simulink model "b_r309c_med"  (Simulink 6.2)
settings: Solver=ode45  StartTime=0.0  StopTime=1030.0  RelTol=1e-3
undefined symbols (not defined in the file): ant_bits, BEE2_usr, blockCountBits, blockRowBits, cmult_4bit_em
libraries: xbsIndex_r3 x2808, xps_library x97, casper_library x84
(part 9 of 20)

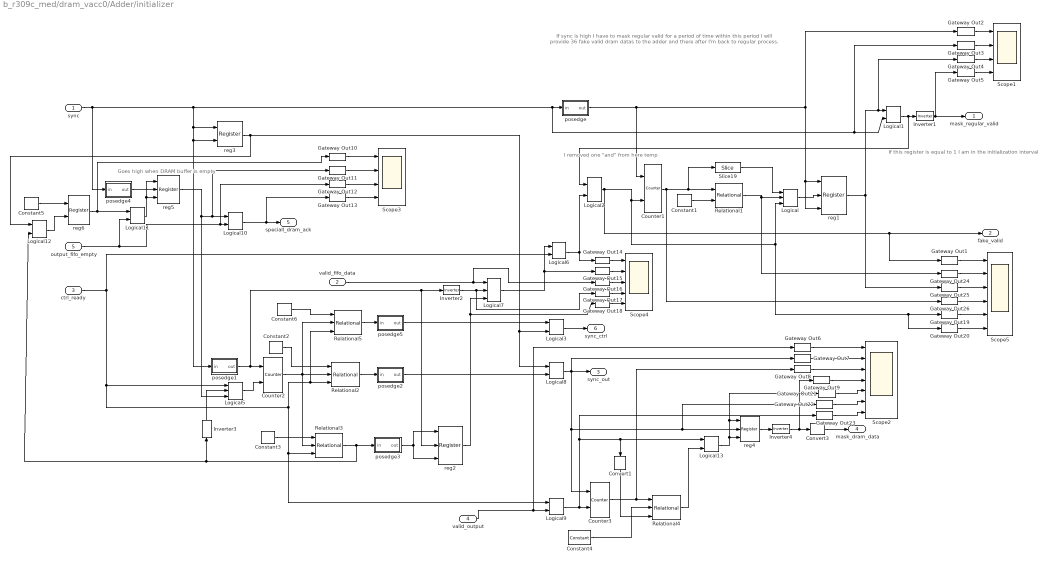
== system b_r309c_med/dram_vacc0/Adder/initializer ==
  note: I removed one "and"
      | from here temp
  note: If this register is equal to 1 I am
      | in the initialization interval
  note: If sync is high I have to mask regular valid for a period of time
      | within this period I will provide 36 fake valid dram datas to the adder and there after I'm back to
      | regular process.
  note: Goes high when DRAM
      | buffer is empty
  sync : Inport  Port=1  LatchInput=off
  valid_fifo_data : Inport  Port=2  LatchInput=off
  ctrl_ready : Inport  Port=3  LatchInput=off
  valid_output : Inport  Port=4  LatchInput=off
  output_fifo_empty : Inport  Port=5  LatchInput=off
  Constant1 : xbsIndex_r3/Constant  const=34  equ=P=C  arith_type=Unsigned  n_bits=6  bin_pt=0  opselect=C  inp2=PCIN>>17  opr=+  inp1=P  carry=CIN  iostate=0  explicit_period=on  period=1  dbl_ovrd=off
  Constant2 : xbsIndex_r3/Constant  const=7  equ=P=C  arith_type=Unsigned  n_bits=4  bin_pt=0  opselect=C  inp2=PCIN>>17  opr=+  inp1=P  carry=CIN  iostate=0  explicit_period=on  period=1  dbl_ovrd=off
  Constant3 : xbsIndex_r3/Constant  const=14  equ=P=C  arith_type=Unsigned  n_bits=4  bin_pt=0  opselect=C  inp2=PCIN>>17  opr=+  inp1=P  carry=CIN  iostate=0  explicit_period=on  period=1  dbl_ovrd=off
  Constant4 : xbsIndex_r3/Constant  const=acc_length-2  equ=P=C  arith_type=Unsigned  n_bits=22  bin_pt=0  opselect=C  inp2=PCIN>>17  opr=+  inp1=P  carry=CIN  iostate=0  explicit_period=on  period=1  dbl_ovrd=off
  Constant5 : xbsIndex_r3/Constant  const=0  equ=P=C  arith_type=Boolean  n_bits=4  bin_pt=0  opselect=C  inp2=PCIN>>17  opr=+  inp1=P  carry=CIN  iostate=0  explicit_period=on  period=1  dbl_ovrd=off
  Constant6 : xbsIndex_r3/Constant  const=4  equ=P=C  arith_type=Unsigned  n_bits=4  bin_pt=0  opselect=C  inp2=PCIN>>17  opr=+  inp1=P  carry=CIN  iostate=0  explicit_period=on  period=1  dbl_ovrd=off
  Convert1 : xbsIndex_r3/Convert  Orientation=down  arith_type=Boolean  n_bits=1  bin_pt=0  quantization=Truncate  overflow=Wrap  latency=0  explicit_period=off  period=1  dbl_ovrd=off  show_param=off  inserted_by_tool=off  pipeline=off
      settings: xl_area=[0, 0, 0, 0, 0, 0, 0]
  Convert3 : xbsIndex_r3/Convert  arith_type=Unsigned  n_bits=1  bin_pt=0  quantization=Truncate  overflow=Wrap  latency=0  explicit_period=off  period=1  dbl_ovrd=off  show_param=off  inserted_by_tool=off  pipeline=off
      settings: xl_area=[0, 0, 0, 0, 0, 0, 0]
  Counter1 : xbsIndex_r3/Counter  cnt_type=Count Limited  n_bits=6  bin_pt=0  arith_type=Unsigned  start_count=0  cnt_to=35  cnt_by_val=1  operation=Up  explicit_period=on  period=1  load_pin=off  rst=on  en=on  dbl_ovrd=off  show_param=off  use_rpm=on  gen_core=off
      settings: xl_area=[0, 0, 0, 0, 0, 0, 0]
  Counter2 : xbsIndex_r3/Counter  cnt_type=Free Running  n_bits=4  bin_pt=0  arith_type=Unsigned  start_count=0  cnt_to=35  cnt_by_val=1  operation=Up  explicit_period=on  period=1  load_pin=off  rst=on  en=on  dbl_ovrd=off  show_param=off  use_rpm=on  gen_core=off
      settings: xl_area=[0, 0, 0, 0, 0, 0, 0]
  Counter3 : xbsIndex_r3/Counter  cnt_type=Free Running  n_bits=22  bin_pt=0  arith_type=Unsigned  start_count=0  cnt_to=35  cnt_by_val=1  operation=Up  explicit_period=on  period=1  load_pin=off  rst=on  en=on  dbl_ovrd=off  show_param=off  use_rpm=on  gen_core=off
      settings: xl_area=[0, 0, 0, 0, 0, 0, 0]
  Gateway Out{1..26} (26 alike) : xbsIndex_r3/Gateway Out  output_type=Double  nbits=8  bin_pt=6  arith_type=Boolean  quantization=Truncate  overflow=Wrap  hdl_port=off  timing_constraint=None  locs_specified=off  LOCs={}  needs_fixed_name=off  show_param=off
      settings: xl_area=[0, 0, 0, 0, 0, 0, 0]
  Inverter1 : xbsIndex_r3/Inverter  latency=0  explicit_period=off  period=1  en=off  dbl_ovrd=off  show_param=off
      settings: xl_area=[0, 0, 0, 0, 0, 0, 0]
  Inverter2 : xbsIndex_r3/Inverter  latency=0  explicit_period=off  period=1  en=off  dbl_ovrd=off  show_param=off
      settings: xl_area=[0, 0, 0, 0, 0, 0, 0]
  Inverter3 : xbsIndex_r3/Inverter  Orientation=up  latency=0  explicit_period=off  period=1  en=off  dbl_ovrd=off  show_param=off
      settings: xl_area=[0, 0, 0, 0, 0, 0, 0]
  Inverter4 : xbsIndex_r3/Inverter  latency=0  explicit_period=off  period=1  en=off  dbl_ovrd=off  show_param=off
      settings: xl_area=[0, 0, 0, 0, 0, 0, 0]
  Logical : xbsIndex_r3/Logical  logical_function=AND  inputs=3  precision=Full  arith_type=Unsigned  n_bits=8  bin_pt=2  align_bp=on  latency=0  explicit_period=on  period=1  en=off  dbl_ovrd=off  show_param=off
      settings: xl_area=[0, 0, 0, 0, 0, 0, 0]
  Logical1 : xbsIndex_r3/Logical  logical_function=OR  inputs=2  precision=Full  arith_type=Unsigned  n_bits=8  bin_pt=2  align_bp=on  latency=0  explicit_period=off  period=1  en=off  dbl_ovrd=off  show_param=off
      settings: xl_area=[0, 0, 0, 0, 0, 0, 0]
  Logical10 : xbsIndex_r3/Logical  logical_function=NOR  inputs=2  precision=Full  arith_type=Unsigned  n_bits=8  bin_pt=2  align_bp=on  latency=0  explicit_period=off  period=1  en=off  dbl_ovrd=off  show_param=off
      settings: xl_area=[0, 0, 0, 0, 0, 0, 0]
  Logical11 : xbsIndex_r3/Logical  logical_function=OR  inputs=2  precision=Full  arith_type=Unsigned  n_bits=8  bin_pt=2  align_bp=on  latency=0  explicit_period=off  period=1  en=off  dbl_ovrd=off  show_param=off
      settings: xl_area=[0, 0, 0, 0, 0, 0, 0]
  Logical{2..3,6,8..9,12..13} (7 alike) : xbsIndex_r3/Logical  logical_function=AND  inputs=2  precision=Full  arith_type=Unsigned  n_bits=8  bin_pt=2  align_bp=on  latency=0  explicit_period=off  period=1  en=off  dbl_ovrd=off  show_param=off
      settings: xl_area=[0, 0, 0, 0, 0, 0, 0]
  Logical5 : xbsIndex_r3/Logical  logical_function=AND  inputs=3  precision=Full  arith_type=Unsigned  n_bits=8  bin_pt=2  align_bp=on  latency=0  explicit_period=off  period=1  en=off  dbl_ovrd=off  show_param=off
      settings: xl_area=[0, 0, 0, 0, 0, 0, 0]
  Logical7 : xbsIndex_r3/Logical  logical_function=AND  inputs=3  precision=Full  arith_type=Unsigned  n_bits=8  bin_pt=2  align_bp=on  latency=0  explicit_period=off  period=1  en=off  dbl_ovrd=off  show_param=off
      settings: xl_area=[0, 0, 0, 0, 0, 0, 0]
  Relational1 : xbsIndex_r3/Relational  mode=a>=b  latency=1  explicit_period=on  period=1  en=off  dbl_ovrd=off  show_param=off
      settings: xl_area=[0, 0, 0, 0, 0, 0, 0]
  Relational2 : xbsIndex_r3/Relational  mode=a<=b  latency=1  explicit_period=on  period=1  en=on  dbl_ovrd=off  show_param=off
      settings: xl_area=[0, 0, 0, 0, 0, 0, 0]
  Relational3 : xbsIndex_r3/Relational  mode=a<=b  latency=1  explicit_period=on  period=1  en=on  dbl_ovrd=off  show_param=off
      settings: xl_area=[0, 0, 0, 0, 0, 0, 0]
  Relational4 : xbsIndex_r3/Relational  mode=a=b  latency=1  explicit_period=on  period=1  en=on  dbl_ovrd=off  show_param=off
      settings: xl_area=[0, 0, 0, 0, 0, 0, 0]
  Relational5 : xbsIndex_r3/Relational  mode=a<=b  latency=1  explicit_period=on  period=1  en=on  dbl_ovrd=off  show_param=off
      settings: xl_area=[0, 0, 0, 0, 0, 0, 0]
  Scope1 : Scope  NumInputPorts=4
      settings: YMin=-1~-1~50~0  YMax=1~1~90~1  SaveName=ScopeData13
  Scope2 : Scope  NumInputPorts=7
      settings: YMin=-1~-1~50~0~-5~-5~-5  YMax=1~1~90~1~5~5~5  SaveName=ScopeData15
  Scope3 : Scope  NumInputPorts=4
      settings: YMin=-1~-1~50~0  YMax=1~1~90~1  SaveName=ScopeData18
  Scope4 : Scope  NumInputPorts=5
      settings: YMin=-1~-1~50~0~-5  YMax=1~1~90~1~5  SaveName=ScopeData31
  Scope5 : Scope  NumInputPorts=6
      settings: YMin=-1~-1~50~0~-5~-5  YMax=1~1~90~1~5~5  SaveName=ScopeData3
  Slice19 : xbsIndex_r3/Slice  mode=Lower Bit Location + Width  nbits=1  bit1=0  base1=MSB of Input  bit0=0  base0=LSB of Input  boolean_output=on  explicit_period=off  period=1  dbl_ovrd=off
  posedge : Subsystem
  posedge1 : Subsystem
  posedge2 : Subsystem
  posedge3 : Subsystem
  posedge4 : Subsystem
  posedge5 : Subsystem
  reg{1..2,4..5} (4 alike) : xbsIndex_r3/Register  init=0  reg_only_valid=off  explicit_period=on  period=1  rst=on  en=on  out_en=off  dbl_ovrd=off  show_param=off
      settings: xl_area=[0, 0, 0, 0, 0, 0, 0]
  reg3 : xbsIndex_r3/Register  init=0  reg_only_valid=off  explicit_period=on  period=1  rst=off  en=on  out_en=off  dbl_ovrd=off  show_param=off
      settings: xl_area=[0, 0, 0, 0, 0, 0, 0]
  reg6 : xbsIndex_r3/Register  init=1  reg_only_valid=off  explicit_period=on  period=1  rst=off  en=on  out_en=off  dbl_ovrd=off  show_param=off
      settings: xl_area=[0, 0, 0, 0, 0, 0, 0]
  mask_regular_valid : Outport
  fake_valid : Outport  Port=2
  sync_out : Outport  Port=3
  mask_dram_data : Outport  Port=4
  speciall_dram_ack : Outport  Port=5
  sync_ctrl : Outport  Port=6
  wires:
  Convert1/1 -> Relational4/3
  Gateway Out23/1 -> Scope2/7
  Gateway Out22/1 -> Scope2/6
  Gateway Out21/1 -> Scope2/5
  Slice19/1 -> Logical/1
  Gateway Out20/1 -> Scope5/6
  Gateway Out19/1 -> Scope5/5
  Gateway Out18/1 -> Scope4/5
  Gateway Out17/1 -> Scope4/4
  Gateway Out16/1 -> Scope4/3
  Gateway Out15/1 -> Scope4/2
  Gateway Out14/1 -> Scope4/1
  Convert3/1 -> mask_dram_data/1
  Relational4/1 -> Logical13/2
  Logical13/1 -> Gateway Out21/1, reg4/1, reg4/3
  reg6/1 -> Gateway Out10/1, Logical11/1
  Logical12/1 -> reg6/2
  Constant5/1 -> reg6/1
  Gateway Out10/1 -> Scope3/1
  Gateway Out13/1 -> Scope3/4
  Gateway Out12/1 -> Scope3/3
  Gateway Out11/1 -> Scope3/2
  Logical11/1 -> reg5/3, reg5/1
  Logical10/1 -> Gateway Out13/1, speciall_dram_ack/1
  output_fifo_empty/1 -> Gateway Out12/1, Logical10/2, Logical11/2
  reg5/1 -> Gateway Out11/1, Logical10/1, Logical5/3
  posedge4/1(out) -> reg5/2
  Gateway Out6/1 -> Scope2/1
  Gateway Out9/1 -> Scope2/4
  Gateway Out8/1 -> Scope2/3
  Gateway Out7/1 -> Scope2/2
  Inverter4/1 -> Convert3/1, Gateway Out9/1
  reg4/1 -> Inverter4/1
  Constant4/1 -> Relational4/2
  Counter3/1 -> Gateway Out8/1, Relational4/1
  valid_output/1 -> Gateway Out6/1, Logical9/2
  Logical9/1 -> Convert1/1, Logical13/1, Gateway Out23/1, Counter3/2
  reg3/1 -> Logical12/1, Logical8/1, Logical3/2
  posedge2/1(out) -> Logical8/2
  Logical8/1 -> Gateway Out7/1, Gateway Out22/1, reg4/2, Counter3/1, sync_out/1
  Inverter3/1 -> Logical5/2
  Logical5/1 -> Counter2/2
  Logical7/1 -> Gateway Out15/1, Logical6/1
  valid_fifo_data/1 -> Gateway Out16/1, Logical7/1
  Inverter2/1 -> Gateway Out17/1, Logical7/2
  reg2/1 -> Gateway Out18/1, Logical7/3
  posedge3/1(out) -> reg2/3, reg2/1
  Relational3/1 -> Logical12/2, Inverter3/1, posedge3/1(in)
  Constant3/1 -> Relational3/1
  Relational2/1 -> posedge2/1(in)
  Constant2/1 -> Relational2/1
  Counter2/1 -> Relational3/2, Relational2/2, Relational5/2
  posedge1/1(out) -> Inverter2/1, reg2/2, Counter2/1
  Inverter1/1 -> Gateway Out5/1, mask_regular_valid/1
  Logical/1 -> reg1/2
  Logical6/1 -> Gateway Out14/1, Logical2/2
  ctrl_ready/1 -> Logical9/1, Relational3/3, Relational2/3, Relational5/3, Logical5/1, Logical6/2
  Relational1/1 -> Logical/2, Gateway Out24/1
  reg1/1 -> Gateway Out25/1, Gateway Out4/1, Logical1/1
  Constant1/1 -> Relational1/2
  Counter1/1 -> Slice19/1, Relational1/1, Gateway Out26/1
  Logical2/1 -> Counter1/2, Gateway Out20/1, Gateway Out19/1, Logical/3, Gateway Out1/1, fake_valid/1
  Logical1/1 -> Logical2/1, Inverter1/1
  posedge/1(out) -> Counter1/1, reg1/3, reg1/1, Gateway Out2/1
  sync/1 -> posedge4/1(in), reg3/1, reg3/2, posedge1/1(in), Gateway Out3/1, Logical1/2, posedge/1(in)
  Gateway Out2/1 -> Scope1/1
  Gateway Out5/1 -> Scope1/4
  Gateway Out4/1 -> Scope1/3
  Gateway Out3/1 -> Scope1/2
  Gateway Out1/1 -> Scope5/1
  Gateway Out26/1 -> Scope5/4
  Gateway Out25/1 -> Scope5/3
  Gateway Out24/1 -> Scope5/2
  Constant6/1 -> Relational5/1
  Relational5/1 -> posedge5/1(in)
  posedge5/1(out) -> Logical3/1
  Logical3/1 -> sync_ctrl/1

== system b_r309c_med/dram_vacc0/RB_reg/Trickle_FWFT ==
  note: We needed a FIFO which brings the valid data automatically to the output.
      | The regular XILINX Fifos are not FWFT (First Word Fall Through).
      | We tried to make one but it was really hard to make one agreeing with the exact specs.
      | This module which we have named it Trickle_FWFT Fifo works very similiarly with minor
      | differences which servers our purpose here in the DRAM VACC module.
  note: The real depth of this module is depth+1.
      | The valid signal will go high with one cycle delay.
  din : Inport  Port=1  LatchInput=off
  we : Inport  Port=2  LatchInput=off
  ack : Inport  Port=3  LatchInput=off
  reset : Inport  Port=4  LatchInput=off
  Convert : xbsIndex_r3/Convert  Orientation=left  arith_type=Boolean  n_bits=8  bin_pt=6  quantization=Truncate  overflow=Wrap  latency=0  explicit_period=on  period=1  dbl_ovrd=off  show_param=off  inserted_by_tool=off  pipeline=off
      settings: xl_area=[0, 0, 0, 0, 0, 0, 0]
  Convert3 : xbsIndex_r3/Convert  arith_type=Boolean  n_bits=8  bin_pt=6  quantization=Truncate  overflow=Wrap  latency=0  explicit_period=off  period=1  dbl_ovrd=off  show_param=off  inserted_by_tool=off  pipeline=off
      settings: xl_area=[0, 0, 0, 0, 0, 0, 0]
  FIFO : xbsIndex_r3/FIFO  depth=16  percent_nbits=1  store_only_valid=on  init_zero=on  explicit_period=on  period=1  rst=on  en=off  use_almost_empty=off  almost_empty_offset=6  use_almost_full=off  almost_full_offset=6  dbl_ovrd=off  show_param=off  mem_type=Block RAM  gen_core=off
      settings: xl_area=[0, 0, 0, 0, 0, 0, 0]
  Inverter3 : xbsIndex_r3/Inverter  latency=0  explicit_period=off  period=1  en=off  dbl_ovrd=off  show_param=off
      settings: xl_area=[0, 0, 0, 0, 0, 0, 0]
  Logical2 : xbsIndex_r3/Logical  logical_function=OR  inputs=2  precision=Full  arith_type=Unsigned  n_bits=8  bin_pt=2  align_bp=on  latency=0  explicit_period=on  period=1  en=off  dbl_ovrd=off  show_param=off
      settings: xl_area=[0, 0, 0, 0, 0, 0, 0]
  not_valid : xbsIndex_r3/Register  init=1  reg_only_valid=off  explicit_period=on  period=1  rst=on  en=on  out_en=off  dbl_ovrd=off  show_param=off
      settings: xl_area=[0, 0, 0, 0, 0, 0, 0]
  data_out : Outport
  valid : Outport  Port=2
  full : Outport  Port=3
  %full : Outport  Port=4
  wires:
  din/1 -> FIFO/1
  we/1 -> FIFO/2
  FIFO/2 -> not_valid/1
  ack/1 -> Logical2/2
  FIFO/1 -> data_out/1
  FIFO/4 -> full/1
  Inverter3/1 -> Convert3/1
  reset/1 -> FIFO/4, not_valid/2
  Logical2/1 -> FIFO/3, not_valid/3
  not_valid/1 -> Inverter3/1, Convert/1
  Convert/1 -> Logical2/1
  FIFO/3 -> %full/1
  Convert3/1 -> valid/1

== system b_r309c_med/dram_vacc0/RB_reg/posedge ==
  in : Inport  Port=1  LatchInput=off
  Delay : xbsIndex_r3/Delay  latency=1  reg_retiming=off  explicit_period=off  period=1  en=off  accept_only_valid=off  init_zero=on  dbl_ovrd=off  show_param=off
      settings: xl_area=[0, 0, 0, 0, 0, 0, 0]
  Inverter2 : xbsIndex_r3/Inverter  latency=0  explicit_period=off  period=1  en=off  dbl_ovrd=off  show_param=off
      settings: xl_area=[0, 0, 0, 0, 0, 0, 0]
  Logical : xbsIndex_r3/Logical  logical_function=AND  inputs=2  precision=Full  arith_type=Unsigned  n_bits=8  bin_pt=2  align_bp=on  latency=0  explicit_period=off  period=1  en=off  dbl_ovrd=off  show_param=off
      settings: xl_area=[0, 0, 0, 0, 0, 0, 0]
  out : Outport
  wires:
  Inverter2/1 -> Logical/1
  Logical/1 -> out/1
  in/1 -> Logical/2, Delay/1
  Delay/1 -> Inverter2/1

== system b_r309c_med/dram_vacc0/ctrl_unit/RB_active_or_finish ==
  enable_rb_addr : Inport  Orientation=down  Port=1  LatchInput=off
  sync : Inport  Port=2  LatchInput=off
  Constant3 : xbsIndex_r3/Constant  const=acc_length/2  equ=P=C  arith_type=Unsigned  n_bits=32  bin_pt=0  opselect=C  inp2=PCIN>>17  opr=+  inp1=P  carry=CIN  iostate=0  explicit_period=on  period=1  dbl_ovrd=off
  Counter1 : xbsIndex_r3/Counter  cnt_type=Free Running  n_bits=32  bin_pt=0  arith_type=Unsigned  start_count=0  cnt_to=2*burst_length-1  cnt_by_val=1  operation=Up  explicit_period=on  period=1  load_pin=off  rst=on  en=on  dbl_ovrd=off  show_param=off  use_rpm=on  gen_core=off
      settings: xl_area=[0, 0, 0, 0, 0, 0, 0]
  Inverter6 : xbsIndex_r3/Inverter  latency=0  explicit_period=off  period=1  en=off  dbl_ovrd=off  show_param=off
      settings: xl_area=[0, 0, 0, 0, 0, 0, 0]
  Inverter9 : xbsIndex_r3/Inverter  latency=0  explicit_period=off  period=1  en=off  dbl_ovrd=off  show_param=off
      settings: xl_area=[0, 0, 0, 0, 0, 0, 0]
  Logical13 : xbsIndex_r3/Logical  logical_function=AND  inputs=3  precision=Full  arith_type=Unsigned  n_bits=8  bin_pt=2  align_bp=on  latency=0  explicit_period=on  period=1  en=off  dbl_ovrd=off  show_param=off
      settings: xl_area=[0, 0, 0, 0, 0, 0, 0]
  Logical14 : xbsIndex_r3/Logical  logical_function=AND  inputs=2  precision=Full  arith_type=Unsigned  n_bits=8  bin_pt=2  align_bp=on  latency=0  explicit_period=on  period=1  en=off  dbl_ovrd=off  show_param=off
      settings: xl_area=[0, 0, 0, 0, 0, 0, 0]
  Logical7 : xbsIndex_r3/Logical  logical_function=AND  inputs=2  precision=Full  arith_type=Unsigned  n_bits=8  bin_pt=2  align_bp=on  latency=0  explicit_period=on  period=1  en=off  dbl_ovrd=off  show_param=off
      settings: xl_area=[0, 0, 0, 0, 0, 0, 0]
  Relational3 : xbsIndex_r3/Relational  mode=a=b  latency=1  explicit_period=on  period=1  en=off  dbl_ovrd=off  show_param=off
      settings: xl_area=[0, 0, 0, 0, 0, 0, 0]
  system_start : xbsIndex_r3/Register  init=0  reg_only_valid=off  explicit_period=off  period=1  rst=off  en=on  out_en=off  dbl_ovrd=off  show_param=off
      settings: xl_area=[0, 0, 0, 0, 0, 0, 0]
  system_start1 : xbsIndex_r3/Register  init=0  reg_only_valid=off  explicit_period=off  period=1  rst=off  en=on  out_en=off  dbl_ovrd=off  show_param=off
      settings: xl_area=[0, 0, 0, 0, 0, 0, 0]
  system_start2 : xbsIndex_r3/Register  init=0  reg_only_valid=off  explicit_period=off  period=1  rst=on  en=on  out_en=off  dbl_ovrd=off  show_param=off
      settings: xl_area=[0, 0, 0, 0, 0, 0, 0]
  rb_active : Outport
  wires:
  Logical13/1 -> rb_active/1
  sync/1 -> system_start2/2, Counter1/1, system_start/2, system_start/1, Logical14/1, Inverter9/1
  enable_rb_addr/1 -> Logical7/1, Counter1/2
  Inverter9/1 -> Logical13/3
  system_start1/1 -> Logical13/2
  Logical14/1 -> system_start1/2, system_start1/1
  Inverter6/1 -> Logical13/1
  Relational3/1 -> Logical7/2
  Logical7/1 -> system_start2/3, system_start2/1
  Constant3/1 -> Relational3/2
  Counter1/1 -> Relational3/1
  system_start2/1 -> Inverter6/1
  system_start/1 -> Logical14/2

== system b_r309c_med/dram_vacc0/ctrl_unit/address_gen_vacc_DRAM ==
  sync : Inport  Port=1  LatchInput=off
  read_en : Inport  Port=2  LatchInput=off
  write_en : Inport  Port=3  LatchInput=off
  and0 : xbsIndex_r3/Logical  logical_function=AND  inputs=2  precision=Full  arith_type=Unsigned  n_bits=8  bin_pt=2  align_bp=on  latency=0  explicit_period=off  period=1  en=off  dbl_ovrd=off  show_param=off
      settings: xl_area=[0, 0, 0, 0, 0, 0, 0]
  block_counter : xbsIndex_r3/Counter  cnt_type=Free Running  n_bits=blockCountBits  bin_pt=0  arith_type=Unsigned  start_count=2^blockCountBits-1  cnt_to=Inf  cnt_by_val=1  operation=Up  explicit_period=off  period=1  load_pin=off  rst=off  en=on  dbl_ovrd=off  show_param=off  use_rpm=on  gen_core=off
      settings: xl_area=[0, 0, 0, 0, 0, 0, 0]
  cast0 : xbsIndex_r3/Convert  arith_type=Unsigned  n_bits=8  bin_pt=0  quantization=Truncate  overflow=Wrap  latency=0  explicit_period=off  period=1  dbl_ovrd=off  show_param=off  inserted_by_tool=off  pipeline=off
      settings: xl_area=[0, 0, 0, 0, 0, 0, 0]
  cast1 : xbsIndex_r3/Convert  arith_type=Unsigned  n_bits=8  bin_pt=0  quantization=Truncate  overflow=Wrap  latency=0  explicit_period=off  period=1  dbl_ovrd=off  show_param=off  inserted_by_tool=off  pipeline=off
      settings: xl_area=[0, 0, 0, 0, 0, 0, 0]
  compare : xbsIndex_r3/Relational  mode=a=b  latency=1  explicit_period=off  period=1  en=off  dbl_ovrd=off  show_param=off
      settings: xl_area=[0, 0, 0, 0, 0, 0, 0]
  compare1 : xbsIndex_r3/Relational  mode=a=b  latency=1  explicit_period=on  period=1  en=off  dbl_ovrd=off  show_param=off
      settings: xl_area=[0, 0, 0, 0, 0, 0, 0]
  concat0 : xbsIndex_r3/Concat  num_inputs=2  explicit_period=off  period=1  dbl_ovrd=off
  concat1 : xbsIndex_r3/Concat  num_inputs=2  explicit_period=off  period=1  dbl_ovrd=off
  concat2 : xbsIndex_r3/Concat  num_inputs=7  explicit_period=off  period=1  dbl_ovrd=off
  concat3 : xbsIndex_r3/Concat  num_inputs=7  explicit_period=off  period=1  dbl_ovrd=off
  const0 : xbsIndex_r3/Constant  const=0  equ=P=C  arith_type=Unsigned  n_bits=5  bin_pt=0  opselect=C  inp2=PCIN>>17  opr=+  inp1=P  carry=CIN  iostate=0  explicit_period=off  period=1  dbl_ovrd=off
  const1 : xbsIndex_r3/Constant  const=0  equ=P=C  arith_type=Unsigned  n_bits=2  bin_pt=0  opselect=C  inp2=PCIN>>17  opr=+  inp1=P  carry=CIN  iostate=0  explicit_period=off  period=1  dbl_ovrd=off
  const10 : xbsIndex_r3/Constant  const=valid_length/2  equ=P=C  arith_type=Unsigned  n_bits=counterBitWidth  bin_pt=0  opselect=C  inp2=PCIN>>17  opr=+  inp1=P  carry=CIN  iostate=0  explicit_period=on  period=1  dbl_ovrd=off
  const11 : xbsIndex_r3/Constant  const=acc_length/2-1  equ=P=C  arith_type=Unsigned  n_bits=counterBitWidth  bin_pt=0  opselect=C  inp2=PCIN>>17  opr=+  inp1=P  carry=CIN  iostate=0  explicit_period=on  period=1  dbl_ovrd=off
  const4 : xbsIndex_r3/Constant  const=acc_length/2-1  equ=P=C  arith_type=Unsigned  n_bits=counterBitWidth  bin_pt=0  opselect=C  inp2=PCIN>>17  opr=+  inp1=P  carry=CIN  iostate=0  explicit_period=off  period=1  dbl_ovrd=off
  or0 : xbsIndex_r3/Logical  logical_function=OR  inputs=2  precision=Full  arith_type=Unsigned  n_bits=8  bin_pt=2  align_bp=on  latency=0  explicit_period=off  period=1  en=off  dbl_ovrd=off  show_param=off
      settings: xl_area=[0, 0, 0, 0, 0, 0, 0]
  read_counter : xbsIndex_r3/Counter  cnt_type=Free Running  n_bits=counterBitWidth  bin_pt=0  arith_type=Unsigned  start_count=0  cnt_to=Inf  cnt_by_val=1  operation=Up  explicit_period=off  period=1  load_pin=on  rst=on  en=on  dbl_ovrd=off  show_param=off  use_rpm=on  gen_core=off
      settings: xl_area=[0, 0, 0, 0, 0, 0, 0]
  slice0 : xbsIndex_r3/Slice  mode=Lower Bit Location + Width  nbits=colCountBits  bit1=0  base1=MSB of Input  bit0=0  base0=LSB of Input  boolean_output=off  explicit_period=off  period=1  dbl_ovrd=off
  slice1 : xbsIndex_r3/Slice  mode=Upper Bit Location + Width  nbits=blockCountBits+blockRowBits  bit1=0  base1=MSB of Input  bit0=0  base0=LSB of Input  boolean_output=off  explicit_period=off  period=1  dbl_ovrd=off
  slice10 : xbsIndex_r3/Slice  mode=Lower Bit Location + Width  nbits=2  bit1=0  base1=MSB of Input  bit0=0  base0=LSB of Input  boolean_output=off  explicit_period=off  period=1  dbl_ovrd=off
  slice11 : xbsIndex_r3/Slice  mode=Upper Bit Location + Width  nbits=blockCountBits-2  bit1=0  base1=MSB of Input  bit0=0  base0=LSB of Input  boolean_output=off  explicit_period=off  period=1  dbl_ovrd=off
  slice12 : xbsIndex_r3/Slice  mode=Upper Bit Location + Width  nbits=1  bit1=0  base1=MSB of Input  bit0=0  base0=LSB of Input  boolean_output=off  explicit_period=off  period=1  dbl_ovrd=off
  slice13 : xbsIndex_r3/Slice  mode=Lower Bit Location + Width  nbits=blockCountBits-3  bit1=0  base1=MSB of Input  bit0=0  base0=LSB of Input  boolean_output=off  explicit_period=off  period=1  dbl_ovrd=off
  slice14 : xbsIndex_r3/Slice  mode=Upper Bit Location + Width  nbits=1  bit1=0  base1=MSB of Input  bit0=0  base0=LSB of Input  boolean_output=off  explicit_period=off  period=1  dbl_ovrd=off
  slice15 : xbsIndex_r3/Slice  mode=Lower Bit Location + Width  nbits=blockCountBits-3  bit1=0  base1=MSB of Input  bit0=0  base0=LSB of Input  boolean_output=off  explicit_period=off  period=1  dbl_ovrd=off
  slice2 : xbsIndex_r3/Slice  mode=Lower Bit Location + Width  nbits=blockRowBits  bit1=0  base1=MSB of Input  bit0=0  base0=LSB of Input  boolean_output=off  explicit_period=off  period=1  dbl_ovrd=off
  slice3 : xbsIndex_r3/Slice  mode=Upper Bit Location + Width  nbits=blockCountBits  bit1=0  base1=MSB of Input  bit0=0  base0=LSB of Input  boolean_output=off  explicit_period=off  period=1  dbl_ovrd=off
  slice4 : xbsIndex_r3/Slice  mode=Lower Bit Location + Width  nbits=2  bit1=0  base1=MSB of Input  bit0=0  base0=LSB of Input  boolean_output=off  explicit_period=off  period=1  dbl_ovrd=off
  slice5 : xbsIndex_r3/Slice  mode=Upper Bit Location + Width  nbits=blockCountBits-2  bit1=0  base1=MSB of Input  bit0=0  base0=LSB of Input  boolean_output=off  explicit_period=off  period=1  dbl_ovrd=off
  slice6 : xbsIndex_r3/Slice  mode=Lower Bit Location + Width  nbits=colCountBits  bit1=0  base1=MSB of Input  bit0=0  base0=LSB of Input  boolean_output=off  explicit_period=off  period=1  dbl_ovrd=off
  slice7 : xbsIndex_r3/Slice  mode=Upper Bit Location + Width  nbits=blockCountBits+blockRowBits  bit1=0  base1=MSB of Input  bit0=0  base0=LSB of Input  boolean_output=off  explicit_period=off  period=1  dbl_ovrd=off
  slice8 : xbsIndex_r3/Slice  mode=Lower Bit Location + Width  nbits=blockRowBits  bit1=0  base1=MSB of Input  bit0=0  base0=LSB of Input  boolean_output=off  explicit_period=off  period=1  dbl_ovrd=off
  slice9 : xbsIndex_r3/Slice  mode=Upper Bit Location + Width  nbits=blockCountBits  bit1=0  base1=MSB of Input  bit0=0  base0=LSB of Input  boolean_output=off  explicit_period=off  period=1  dbl_ovrd=off
  write_counter : xbsIndex_r3/Counter  cnt_type=Count Limited  n_bits=counterBitWidth  bin_pt=0  arith_type=Unsigned  start_count=0  cnt_to=acc_length/2-1  cnt_by_val=1  operation=Up  explicit_period=off  period=1  load_pin=off  rst=on  en=on  dbl_ovrd=off  show_param=off  use_rpm=on  gen_core=off
      settings: xl_area=[0, 0, 0, 0, 0, 0, 0]
  write_addr : Outport
  read_addr : Outport  Port=2
  end_masking : Outport  Port=3
  wires:
  slice1/1 -> slice2/1, slice3/1
  const1/1 -> concat2/1, concat3/1
  slice4/1 -> concat2/2
  slice13/1 -> concat2/3
  slice2/1 -> concat2/4
  slice12/1 -> concat2/5
  cast0/1 -> concat2/6
  const0/1 -> concat2/7, concat3/7
  slice7/1 -> slice8/1, slice9/1
  slice10/1 -> concat3/2
  slice15/1 -> concat3/3
  slice8/1 -> concat3/4
  slice14/1 -> concat3/5
  cast1/1 -> concat3/6
  sync/1 -> write_counter/1, read_counter/1, block_counter/1, or0/1
  const10/1 -> read_counter/2
  write_en/1 -> write_counter/2
  block_counter/1 -> concat0/1, concat1/1
  write_counter/1 -> concat0/2, compare/1
  read_counter/1 -> concat1/2, compare1/1
  const4/1 -> compare/2
  compare/1 -> end_masking/1
  const11/1 -> compare1/2
  concat0/1 -> slice0/1, slice1/1
  slice0/1 -> cast0/1
  slice3/1 -> slice4/1, slice5/1
  concat2/1 -> write_addr/1
  concat1/1 -> slice6/1, slice7/1
  slice6/1 -> cast1/1
  slice9/1 -> slice10/1, slice11/1
  concat3/1 -> read_addr/1
  slice5/1 -> slice12/1, slice13/1
  slice11/1 -> slice14/1, slice15/1
  read_en/1 -> or0/2, and0/1
  or0/1 -> read_counter/4
  compare1/1 -> and0/2
  and0/1 -> read_counter/3

== system b_r309c_med/dram_vacc0/ctrl_unit/cmd_gen ==
  note: Logic here is added to handle an  odd number of input valid datas.
      | In case we receive a new sync and valid_wr_cnt is high, we mask the wr_be
      | signal of DRAM and issue a write command to finish the last command.
  valid_data : Inport  Port=1  LatchInput=off
  sync : Inport  Port=2  LatchInput=off
  Constant : xbsIndex_r3/Constant  const=burst_length-1  equ=P=C  arith_type=Unsigned  n_bits=ceil(log2(2*burst_length+2))  bin_pt=0  opselect=C  inp2=PCIN>>17  opr=+  inp1=P  carry=CIN  iostate=0  explicit_period=on  period=1  dbl_ovrd=off
  Constant1 : xbsIndex_r3/Constant  const=burst_length-1  equ=P=C  arith_type=Unsigned  n_bits=ceil(log2(2*burst_length+2))  bin_pt=0  opselect=C  inp2=PCIN>>17  opr=+  inp1=P  carry=CIN  iostate=0  explicit_period=on  period=1  dbl_ovrd=off
  Constant2 : xbsIndex_r3/Constant  const=2*burst_length+2-1  equ=P=C  arith_type=Unsigned  n_bits=ceil(log2(2*burst_length+2))  bin_pt=0  opselect=C  inp2=PCIN>>17  opr=+  inp1=P  carry=CIN  iostate=0  explicit_period=on  period=1  dbl_ovrd=off
  Constant3 : xbsIndex_r3/Constant  const=2^18-1  equ=P=C  arith_type=Unsigned  n_bits=18  bin_pt=0  opselect=C  inp2=PCIN>>17  opr=+  inp1=P  carry=CIN  iostate=0  explicit_period=on  period=1  dbl_ovrd=off
  Constant4 : xbsIndex_r3/Constant  const=2*burst_length  equ=P=C  arith_type=Unsigned  n_bits=ceil(log2(2*burst_length+2))  bin_pt=0  opselect=C  inp2=PCIN>>17  opr=+  inp1=P  carry=CIN  iostate=0  explicit_period=on  period=1  dbl_ovrd=off
  Convert1 : xbsIndex_r3/Convert  arith_type=Boolean  n_bits=31  bin_pt=0  quantization=Truncate  overflow=Wrap  latency=0  explicit_period=on  period=1  dbl_ovrd=off  show_param=off  inserted_by_tool=off  pipeline=off
      settings: xl_area=[0, 0, 0, 0, 0, 0, 0]
  Delay : xbsIndex_r3/Delay  latency=1  reg_retiming=off  explicit_period=off  period=1  en=on  accept_only_valid=off  init_zero=on  dbl_ovrd=off  show_param=off
      settings: xl_area=[0, 0, 0, 0, 0, 0, 0]
  Delay1 : xbsIndex_r3/Delay  latency=1  reg_retiming=off  explicit_period=off  period=1  en=off  accept_only_valid=off  init_zero=on  dbl_ovrd=off  show_param=off
      settings: xl_area=[0, 0, 0, 0, 0, 0, 0]
  Delay3 : xbsIndex_r3/Delay  latency=1  reg_retiming=off  explicit_period=on  period=1  en=off  accept_only_valid=off  init_zero=on  dbl_ovrd=off  show_param=off
      settings: xl_area=[0, 0, 0, 0, 0, 0, 0]
  Delay4 : xbsIndex_r3/Delay  latency=1  reg_retiming=off  explicit_period=on  period=1  en=off  accept_only_valid=off  init_zero=on  dbl_ovrd=off  show_param=off
      settings: xl_area=[0, 0, 0, 0, 0, 0, 0]
  Inverter{1..5} (5 alike) : xbsIndex_r3/Inverter  latency=0  explicit_period=off  period=1  en=off  dbl_ovrd=off  show_param=off
      settings: xl_area=[0, 0, 0, 0, 0, 0, 0]
  Inverter8 : xbsIndex_r3/Inverter  Orientation=down  latency=0  explicit_period=off  period=1  en=off  dbl_ovrd=off  show_param=off
      settings: xl_area=[0, 0, 0, 0, 0, 0, 0]
  Logical{,2,8..9,12,15} (6 alike) : xbsIndex_r3/Logical  logical_function=AND  inputs=2  precision=Full  arith_type=Unsigned  n_bits=8  bin_pt=2  align_bp=on  latency=0  explicit_period=on  period=1  en=off  dbl_ovrd=off  show_param=off
      settings: xl_area=[0, 0, 0, 0, 0, 0, 0]
  Logical1 : xbsIndex_r3/Logical  logical_function=AND  inputs=3  precision=Full  arith_type=Unsigned  n_bits=8  bin_pt=2  align_bp=on  latency=0  explicit_period=on  period=1  en=off  dbl_ovrd=off  show_param=off
      settings: xl_area=[0, 0, 0, 0, 0, 0, 0]
  Logical10 : xbsIndex_r3/Logical  logical_function=OR  inputs=2  precision=Full  arith_type=Unsigned  n_bits=8  bin_pt=2  align_bp=on  latency=0  explicit_period=on  period=1  en=off  dbl_ovrd=off  show_param=off
      settings: xl_area=[0, 0, 0, 0, 0, 0, 0]
  Logical11 : xbsIndex_r3/Logical  logical_function=OR  inputs=2  precision=Full  arith_type=Unsigned  n_bits=8  bin_pt=2  align_bp=on  latency=0  explicit_period=on  period=1  en=off  dbl_ovrd=off  show_param=off
      settings: xl_area=[0, 0, 0, 0, 0, 0, 0]
  Logical3 : xbsIndex_r3/Logical  logical_function=AND  inputs=3  precision=Full  arith_type=Unsigned  n_bits=8  bin_pt=2  align_bp=on  latency=0  explicit_period=off  period=1  en=off  dbl_ovrd=off  show_param=off
      settings: xl_area=[0, 0, 0, 0, 0, 0, 0]
  Logical4 : xbsIndex_r3/Logical  logical_function=OR  inputs=2  precision=Full  arith_type=Unsigned  n_bits=8  bin_pt=2  align_bp=on  latency=0  explicit_period=off  period=1  en=off  dbl_ovrd=off  show_param=off
      settings: xl_area=[0, 0, 0, 0, 0, 0, 0]
  Logical5 : xbsIndex_r3/Logical  logical_function=OR  inputs=2  precision=Full  arith_type=Unsigned  n_bits=8  bin_pt=2  align_bp=on  latency=0  explicit_period=off  period=1  en=off  dbl_ovrd=off  show_param=off
      settings: xl_area=[0, 0, 0, 0, 0, 0, 0]
  Logical6 : xbsIndex_r3/Logical  logical_function=OR  inputs=2  precision=Full  arith_type=Unsigned  n_bits=8  bin_pt=2  align_bp=on  latency=0  explicit_period=on  period=1  en=off  dbl_ovrd=off  show_param=off
      settings: xl_area=[0, 0, 0, 0, 0, 0, 0]
  Relational : xbsIndex_r3/Relational  mode=a>=b  latency=1  explicit_period=on  period=1  en=on  dbl_ovrd=off  show_param=off
      settings: xl_area=[0, 0, 0, 0, 0, 0, 0]
  Relational1 : xbsIndex_r3/Relational  mode=a<=b  latency=1  explicit_period=on  period=1  en=on  dbl_ovrd=off  show_param=off
      settings: xl_area=[0, 0, 0, 0, 0, 0, 0]
  Relational2 : xbsIndex_r3/Relational  mode=a!=b  latency=1  explicit_period=off  period=1  en=on  dbl_ovrd=off  show_param=off
      settings: xl_area=[0, 0, 0, 0, 0, 0, 0]
  Relational4 : xbsIndex_r3/Relational  mode=a<=b  latency=1  explicit_period=on  period=1  en=on  dbl_ovrd=off  show_param=off
      settings: xl_area=[0, 0, 0, 0, 0, 0, 0]
  Slice : xbsIndex_r3/Slice  mode=Lower Bit Location + Width  nbits=1  bit1=0  base1=MSB of Input  bit0=0  base0=LSB of Input  boolean_output=on  explicit_period=off  period=1  dbl_ovrd=off
  cmd_counter : xbsIndex_r3/Counter  cnt_type=Count Limited  n_bits=ceil(log2(2*burst_length+2))  bin_pt=0  arith_type=Unsigned  start_count=0  cnt_to=2*burst_length+2-1  cnt_by_val=1  operation=Up  explicit_period=on  period=1  load_pin=off  rst=on  en=on  dbl_ovrd=off  show_param=off  use_rpm=on  gen_core=off
      settings: xl_area=[0, 0, 0, 0, 0, 0, 0]
  system_start : xbsIndex_r3/Register  init=0  reg_only_valid=off  explicit_period=off  period=1  rst=off  en=on  out_en=off  dbl_ovrd=off  show_param=off
      settings: xl_area=[0, 0, 0, 0, 0, 0, 0]
  re_addr_en : Outport
  wr_addr_en : Outport  Port=2
  RWn : Outport  Port=3
  cmd_valid : Outport  Port=4
  ready : Outport  Port=5
  rb_addr_en : Outport  Port=6
  wr_be : Outport  Port=7
  wires:
  Logical9/1 -> wr_addr_en/1
  Logical8/1 -> re_addr_en/1
  Logical15/1 -> Logical4/1, Logical11/1
  Inverter8/1 -> Logical1/3
  Relational4/1 -> rb_addr_en/1, Inverter8/1
  Constant4/1 -> Relational4/1
  Logical6/1 -> Delay/2, Relational4/3, Relational/3, Relational1/3, Relational2/3
  Delay4/1 -> Logical6/1, Logical5/2
  Logical5/1 -> cmd_counter/1
  Logical2/1 -> Delay3/1
  Logical12/1 -> Logical2/1
  Convert1/1 -> Logical2/2, Logical8/2, Logical9/2, Logical6/2
  Inverter5/1 -> Logical15/2, ready/1
  Inverter4/1 -> Logical10/1
  Logical10/1 -> Logical12/1
  Inverter3/1 -> RWn/1
  Inverter2/1 -> Logical1/2
  system_start/1 -> Logical12/2
  Logical4/1 -> cmd_counter/2
  Logical3/1 -> Logical11/2, Logical4/2, Inverter5/1
  valid_data/1 -> Logical15/1
  Delay1/1 -> Inverter1/1
  Inverter1/1 -> Logical3/2
  Relational2/1 -> Logical3/3
  Constant2/1 -> Relational2/1
  Relational1/1 -> Logical3/1
  Constant1/1 -> Relational1/1
  Delay/1 -> Logical/1, Logical1/1
  Relational/1 -> Inverter3/1, Logical10/2, Logical/2, Inverter2/1
  Slice/1 -> Inverter4/1, Delay/1
  Logical1/1 -> Logical8/1
  Logical/1 -> Logical9/1
  Logical11/1 -> Convert1/1
  Constant/1 -> Relational/1
  cmd_counter/1 -> Relational2/2, Relational1/2, Relational4/2, Relational/2, Slice/1
  sync/1 -> Delay4/1, Logical5/1, system_start/1, system_start/2, Delay1/1
  Constant3/1 -> wr_be/1
  Delay3/1 -> cmd_valid/1

== system b_r309c_med/dram_vacc0/ctrl_unit/latch_rb_enable ==
  sync : Inport  Port=1  LatchInput=off
  rb_addr_enable : Inport  Port=2  LatchInput=off
  negedge : Inport  Port=3  LatchInput=off
  Inverter5 : xbsIndex_r3/Inverter  latency=0  explicit_period=off  period=1  en=off  dbl_ovrd=off  show_param=off
      settings: xl_area=[0, 0, 0, 0, 0, 0, 0]
  Logical1 : xbsIndex_r3/Logical  logical_function=OR  inputs=2  precision=Full  arith_type=Unsigned  n_bits=8  bin_pt=2  align_bp=on  latency=0  explicit_period=on  period=1  en=off  dbl_ovrd=off  show_param=off
      settings: xl_area=[0, 0, 0, 0, 0, 0, 0]
  Logical2 : xbsIndex_r3/Logical  logical_function=OR  inputs=2  precision=Full  arith_type=Unsigned  n_bits=8  bin_pt=2  align_bp=on  latency=1  explicit_period=on  period=1  en=off  dbl_ovrd=off  show_param=off
      settings: xl_area=[0, 0, 0, 0, 0, 0, 0]
  Logical3 : xbsIndex_r3/Logical  logical_function=AND  inputs=2  precision=Full  arith_type=Unsigned  n_bits=8  bin_pt=2  align_bp=on  latency=0  explicit_period=on  period=1  en=off  dbl_ovrd=off  show_param=off
      settings: xl_area=[0, 0, 0, 0, 0, 0, 0]
  Logical4 : xbsIndex_r3/Logical  logical_function=AND  inputs=2  precision=Full  arith_type=Unsigned  n_bits=8  bin_pt=2  align_bp=on  latency=0  explicit_period=on  period=1  en=off  dbl_ovrd=off  show_param=off
      settings: xl_area=[0, 0, 0, 0, 0, 0, 0]
  system_start3 : xbsIndex_r3/Register  init=0  reg_only_valid=off  explicit_period=off  period=1  rst=off  en=on  out_en=off  dbl_ovrd=off  show_param=off
      settings: xl_area=[0, 0, 0, 0, 0, 0, 0]
  inc_addr_en : Outport
  cmd_tag : Outport  Port=2
  wires:
  Inverter5/1 -> Logical4/2
  Logical3/1 -> inc_addr_en/1
  negedge/1 -> system_start3/2, Logical3/2, Inverter5/1
  rb_addr_enable/1 -> Logical1/2
  sync/1 -> Logical1/1
  Logical4/1 -> Logical2/1
  Logical2/1 -> Logical4/1, system_start3/1
  Logical1/1 -> Logical2/2
  system_start3/1 -> cmd_tag/1, Logical3/1

== system b_r309c_med/dram_vacc0/ctrl_unit/negedge ==
  in : Inport  Port=1  LatchInput=off
  Delay : xbsIndex_r3/Delay  latency=1  reg_retiming=off  explicit_period=off  period=1  en=off  accept_only_valid=off  init_zero=on  dbl_ovrd=off  show_param=off
      settings: xl_area=[0, 0, 0, 0, 0, 0, 0]
  Inverter1 : xbsIndex_r3/Inverter  latency=0  explicit_period=off  period=1  en=off  dbl_ovrd=off  show_param=off
      settings: xl_area=[0, 0, 0, 0, 0, 0, 0]
  Logical : xbsIndex_r3/Logical  logical_function=AND  inputs=2  precision=Full  arith_type=Unsigned  n_bits=8  bin_pt=2  align_bp=on  latency=0  explicit_period=off  period=1  en=off  dbl_ovrd=off  show_param=off
      settings: xl_area=[0, 0, 0, 0, 0, 0, 0]
  out : Outport
  wires:
  Inverter1/1 -> Logical/2
  Delay/1 -> Logical/1
  in/1 -> Inverter1/1, Delay/1
  Logical/1 -> out/1

== system b_r309c_med/dram_vacc0/ctrl_unit/readback_address_dram_vacc ==
  sync : Inport  Port=1  LatchInput=off
  en : Inport  Port=2  LatchInput=off
  block_counter : xbsIndex_r3/Counter  cnt_type=Free Running  n_bits=blockCountBits  bin_pt=0  arith_type=Unsigned  start_count=2^blockCountBits-2  cnt_to=Inf  cnt_by_val=1  operation=Up  explicit_period=off  period=1  load_pin=off  rst=off  en=on  dbl_ovrd=off  show_param=off  use_rpm=on  gen_core=off
      settings: xl_area=[0, 0, 0, 0, 0, 0, 0]
  cast1 : xbsIndex_r3/Convert  arith_type=Unsigned  n_bits=8  bin_pt=0  quantization=Truncate  overflow=Wrap  latency=0  explicit_period=off  period=1  dbl_ovrd=off  show_param=off  inserted_by_tool=off  pipeline=off
      settings: xl_area=[0, 0, 0, 0, 0, 0, 0]
  concat1 : xbsIndex_r3/Concat  num_inputs=2  explicit_period=off  period=1  dbl_ovrd=off
  concat3 : xbsIndex_r3/Concat  num_inputs=7  explicit_period=off  period=1  dbl_ovrd=off
  const0 : xbsIndex_r3/Constant  const=0  equ=P=C  arith_type=Unsigned  n_bits=5  bin_pt=0  opselect=C  inp2=PCIN>>17  opr=+  inp1=P  carry=CIN  iostate=0  explicit_period=off  period=1  dbl_ovrd=off
  const1 : xbsIndex_r3/Constant  const=0  equ=P=C  arith_type=Unsigned  n_bits=2  bin_pt=0  opselect=C  inp2=PCIN>>17  opr=+  inp1=P  carry=CIN  iostate=0  explicit_period=off  period=1  dbl_ovrd=off
  read_counter : xbsIndex_r3/Counter  cnt_type=Count Limited  n_bits=counterBitWidth  bin_pt=0  arith_type=Unsigned  start_count=0  cnt_to=acc_length/2-1  cnt_by_val=1  operation=Up  explicit_period=off  period=1  load_pin=on  rst=on  en=on  dbl_ovrd=off  show_param=off  use_rpm=on  gen_core=off
      settings: xl_area=[0, 0, 0, 0, 0, 0, 0]
  slice10 : xbsIndex_r3/Slice  mode=Lower Bit Location + Width  nbits=2  bit1=0  base1=MSB of Input  bit0=0  base0=LSB of Input  boolean_output=off  explicit_period=off  period=1  dbl_ovrd=off
  slice11 : xbsIndex_r3/Slice  mode=Upper Bit Location + Width  nbits=blockCountBits-2  bit1=0  base1=MSB of Input  bit0=0  base0=LSB of Input  boolean_output=off  explicit_period=off  period=1  dbl_ovrd=off
  slice14 : xbsIndex_r3/Slice  mode=Upper Bit Location + Width  nbits=1  bit1=0  base1=MSB of Input  bit0=0  base0=LSB of Input  boolean_output=off  explicit_period=off  period=1  dbl_ovrd=off
  slice15 : xbsIndex_r3/Slice  mode=Lower Bit Location + Width  nbits=blockCountBits-3  bit1=0  base1=MSB of Input  bit0=0  base0=LSB of Input  boolean_output=off  explicit_period=off  period=1  dbl_ovrd=off
  slice6 : xbsIndex_r3/Slice  mode=Lower Bit Location + Width  nbits=colCountBits  bit1=0  base1=MSB of Input  bit0=0  base0=LSB of Input  boolean_output=off  explicit_period=off  period=1  dbl_ovrd=off
  slice7 : xbsIndex_r3/Slice  mode=Upper Bit Location + Width  nbits=blockCountBits+blockRowBits  bit1=0  base1=MSB of Input  bit0=0  base0=LSB of Input  boolean_output=off  explicit_period=off  period=1  dbl_ovrd=off
  slice8 : xbsIndex_r3/Slice  mode=Lower Bit Location + Width  nbits=blockRowBits  bit1=0  base1=MSB of Input  bit0=0  base0=LSB of Input  boolean_output=off  explicit_period=off  period=1  dbl_ovrd=off
  slice9 : xbsIndex_r3/Slice  mode=Upper Bit Location + Width  nbits=blockCountBits  bit1=0  base1=MSB of Input  bit0=0  base0=LSB of Input  boolean_output=off  explicit_period=off  period=1  dbl_ovrd=off
  readback_addr : Outport
  wires:
  slice7/1 -> slice8/1, slice9/1
  const1/1 -> concat3/1
  slice10/1 -> concat3/2
  slice15/1 -> concat3/3
  slice8/1 -> concat3/4
  slice14/1 -> concat3/5
  cast1/1 -> concat3/6
  const0/1 -> concat3/7
  sync/1 -> read_counter/1, block_counter/1
  en/1 -> read_counter/2
  block_counter/1 -> concat1/1
  read_counter/1 -> concat1/2
  concat1/1 -> slice6/1, slice7/1
  slice6/1 -> cast1/1
  slice9/1 -> slice10/1, slice11/1
  concat3/1 -> readback_addr/1
  slice11/1 -> slice14/1, slice15/1

== system b_r309c_med/dram_vacc0/dram1/sim_wrapper ==
  rst : Inport  Port=1  LatchInput=off
  address : Inport  Port=2  LatchInput=off
  data_in : Inport  Port=3  LatchInput=off
  wr_be : Inport  Port=4  LatchInput=off
  RWn : Inport  Port=5  LatchInput=off
  cmd_tag : Inport  Port=6  LatchInput=off
  cmd_valid : Inport  Port=7  LatchInput=off
  rd_ack : Inport  Port=8  LatchInput=off
  Disregard Subsystem : xbsIndex_r3/Disregard Subsystem  Tag=discardX
      settings: AttributesFormatString=Disregard Subsystem\nFor Generation
  ModelSim : xbsIndex_r3/ModelSim  dir=./modelsim  waveform=on  leave_open=on  skip_compile=off  custom_scripts=off  post_vsim_script=dram_sim.do  startup_timeout=600
  Terminator : Terminator
  Terminator1 : Terminator
  dram_sim : xbsIndex_r3/Black Box  init_code=dram_sim  sim_method=Use HDL Co-Simulation  engine_block=../../../ModelSim  show_param=off
      settings: xl_area=[0, 0, 0, 0, 0, 0, 0]
  cmd_ack : Outport
  data_out : Outport  Port=2
  rd_tag : Outport  Port=3
  rd_valid : Outport  Port=4
  wires:
  rst/1 -> dram_sim/1
  dram_sim/1 -> cmd_ack/1
  dram_sim/2 -> data_out/1
  dram_sim/3 -> rd_tag/1
  dram_sim/4 -> rd_valid/1
  dram_sim/5 -> Terminator/1
  dram_sim/6 -> Terminator1/1
  address/1 -> dram_sim/2
  data_in/1 -> dram_sim/3
  wr_be/1 -> dram_sim/4
  RWn/1 -> dram_sim/5
  cmd_tag/1 -> dram_sim/6
  cmd_valid/1 -> dram_sim/7
  rd_ack/1 -> dram_sim/8

== system b_r309c_med/dram_vacc0/fifo_empty_check/negedge ==
  in : Inport  Port=1  LatchInput=off
  Delay : xbsIndex_r3/Delay  latency=1  reg_retiming=off  explicit_period=off  period=1  en=off  accept_only_valid=off  init_zero=on  dbl_ovrd=off  show_param=off
      settings: xl_area=[0, 0, 0, 0, 0, 0, 0]
  Inverter1 : xbsIndex_r3/Inverter  latency=0  explicit_period=off  period=1  en=off  dbl_ovrd=off  show_param=off
      settings: xl_area=[0, 0, 0, 0, 0, 0, 0]
  Logical : xbsIndex_r3/Logical  logical_function=AND  inputs=2  precision=Full  arith_type=Unsigned  n_bits=8  bin_pt=2  align_bp=on  latency=0  explicit_period=off  period=1  en=off  dbl_ovrd=off  show_param=off
      settings: xl_area=[0, 0, 0, 0, 0, 0, 0]
  out : Outport
  wires:
  Inverter1/1 -> Logical/2
  Logical/1 -> out/1
  in/1 -> Inverter1/1, Delay/1
  Delay/1 -> Logical/1

== system b_r309c_med/loopback0/rollback_fifo/set_cnt ==
  set : Inport  Port=1  LatchInput=off
  undo : Inport  Port=2  LatchInput=off
  en : Inport  Port=3  LatchInput=off
  Counter4 : xbsIndex_r3/Counter  cnt_type=Free Running  n_bits=depth_bits + 1  bin_pt=0  arith_type=Unsigned  start_count=0  cnt_to=Inf  cnt_by_val=1  operation=Up  explicit_period=on  period=1  load_pin=on  rst=off  en=on  dbl_ovrd=off  show_param=off  use_rpm=on  gen_core=off
      settings: xl_area=[0, 0, 0, 0, 0, 0, 0]
  Inverter : xbsIndex_r3/Inverter  latency=0  explicit_period=off  period=1  en=off  dbl_ovrd=off  show_param=off
      settings: xl_area=[0, 0, 0, 0, 0, 0, 0]
  Inverter1 : xbsIndex_r3/Inverter  latency=0  explicit_period=off  period=1  en=off  dbl_ovrd=off  show_param=off
      settings: xl_area=[0, 0, 0, 0, 0, 0, 0]
  Logical1 : xbsIndex_r3/Logical  logical_function=AND  inputs=3  precision=Full  arith_type=Unsigned  n_bits=8  bin_pt=2  align_bp=on  latency=0  explicit_period=off  period=1  en=off  dbl_ovrd=off  show_param=off
      settings: xl_area=[0, 0, 0, 0, 0, 0, 0]
  Logical4 : xbsIndex_r3/Logical  logical_function=AND  inputs=3  precision=Full  arith_type=Unsigned  n_bits=8  bin_pt=2  align_bp=on  latency=1  explicit_period=off  period=1  en=off  dbl_ovrd=off  show_param=off
      settings: xl_area=[0, 0, 0, 0, 0, 0, 0]
  Register2 : xbsIndex_r3/Register  init=0  reg_only_valid=off  explicit_period=off  period=1  rst=off  en=on  out_en=off  dbl_ovrd=off  show_param=off
      settings: xl_area=[0, 0, 0, 0, 0, 0, 0]
  set_cnt : Outport
  cnt : Outport  Port=2
  wires:
  Inverter1/1 -> Logical1/3
  Inverter/1 -> Logical4/3
  undo/1 -> Inverter/1, Logical1/1
  Logical1/1 -> Counter4/1
  set/1 -> Logical4/1
  Logical4/1 -> Inverter1/1, Register2/2
  Register2/1 -> set_cnt/1, Counter4/2
  en/1 -> Logical4/2, Logical1/2, Counter4/3
  Counter4/1 -> Register2/1, cnt/1

== system b_r309c_med/win_x_engine0/auto_tap/a_loop_delay ==
  In1 : Inport  Port=1  LatchInput=off
  delay_bram : casper_library/Delays/delay_bram  DelayLen=(acc_len - 1)*ceil(n_ants/2) + ceil(n_ants/2)-floor(n_ants/2)  bram_latency=bram_latency
  Out1 : Outport
  wires:
  In1/1 -> delay_bram/1
  delay_bram/1 -> Out1/1
